simulink model "fullbridge1ph_igbt_model"  (R2026a)
settings: Solver=ode23t  StopTime=simStopTime
model workspace (MAT data in the model file):
  Cies_IGBT = 5.1e-09
  Cies_IGBT_nF = 5.1
  Cies_IGBT_pF = 5100
  Coes_IGBT = 1e-09
  Coes_IGBT_nF = 1
  Coes_IGBT_pF = 1000
  Cres_IGBT = 3e-10
  Cres_IGBT_nF = 0.3
  Cres_IGBT_pF = 300
  Eoff_sw = 0.0038
  Eon_sw = 0.009
  Eref_I_IGBT = 75
  Eref_T_IGBT = 125
  Eref_V_IGBT = 600
  Ic_VceSat = 75
  Ices = 0.005
  Tmeas_IGBT = 25
  VCE0_IGBT = 1.54
  VceSat = 3.85
  Vces_Ices = 1200
  VgeTh = 5.5
  Vge_VceSat = 15
  Vth = 5.5
  Vth_sw = 5.5
  rCE_IGBT = 0.0308
undefined symbols (not defined in the file): deadSamples, fout, fsw, ModIndex, Rload, Ts_ctrl, Vg
libraries: nesl_utility x28, fl_lib x27, ee_lib x15, simulink x1
(part 2 of 2)

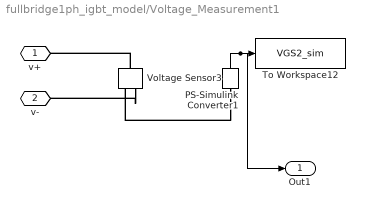
== system fullbridge1ph_igbt_model/Voltage_Measurement1 ==
  PS-Simulink Converter1 : nesl_utility/PS-Simulink Converter  PhysicalDomain=network_engine_domain  SubClassName=ps_output  LeftPortType=input  RightPortType=output  PseudoPeriodic=off  Frequencies=[]  VectorFormat=inherit  Unit=inherit  AffineConversion=off
  To Workspace12 : ToWorkspace  VariableName=VGS2_sim  SaveFormat=Timeseries  SampleTime=-1
  Voltage Sensor3 : fl_lib/Electrical/Electrical Sensors/Voltage Sensor
  v+ : PMIOPort  Side=Left
  v- : PMIOPort  Port=2  Side=Left
  Out1 : Outport
  wires:
  PS-Simulink Converter1/1 -> Out1/1, To Workspace12/1
  connections:
  Voltage Sensor3/RConn2 -- v-/RConn1
  PS-Simulink Converter1/LConn1 -- Voltage Sensor3/RConn1
  Voltage Sensor3/LConn1 -- v+/RConn1

== system fullbridge1ph_igbt_model/Voltage_Measurement2 ==
  PS-Simulink Converter1 : nesl_utility/PS-Simulink Converter  PhysicalDomain=network_engine_domain  SubClassName=ps_output  LeftPortType=input  RightPortType=output  PseudoPeriodic=off  Frequencies=[]  VectorFormat=inherit  Unit=inherit  AffineConversion=off
  To Workspace12 : ToWorkspace  VariableName=VGS1_sim  SaveFormat=Timeseries  SampleTime=-1
  Voltage Sensor3 : fl_lib/Electrical/Electrical Sensors/Voltage Sensor
  v+ : PMIOPort  Side=Left
  v- : PMIOPort  Port=2  Side=Left
  Out1 : Outport
  wires:
  PS-Simulink Converter1/1 -> Out1/1, To Workspace12/1
  connections:
  Voltage Sensor3/RConn2 -- v-/RConn1
  PS-Simulink Converter1/LConn1 -- Voltage Sensor3/RConn1
  Voltage Sensor3/LConn1 -- v+/RConn1

== system fullbridge1ph_igbt_model/Voltage_Measurement3 ==
  PS-Simulink Converter1 : nesl_utility/PS-Simulink Converter  PhysicalDomain=network_engine_domain  SubClassName=ps_output  LeftPortType=input  RightPortType=output  PseudoPeriodic=off  Frequencies=[]  VectorFormat=inherit  Unit=inherit  AffineConversion=off
  To Workspace12 : ToWorkspace  VariableName=VGS3_sim  SaveFormat=Timeseries  SampleTime=-1
  Voltage Sensor3 : fl_lib/Electrical/Electrical Sensors/Voltage Sensor
  v+ : PMIOPort  Side=Left
  v- : PMIOPort  Port=2  Side=Left
  wires:
  PS-Simulink Converter1/1 -> To Workspace12/1
  connections:
  Voltage Sensor3/RConn2 -- v-/RConn1
  PS-Simulink Converter1/LConn1 -- Voltage Sensor3/RConn1
  Voltage Sensor3/LConn1 -- v+/RConn1

== system fullbridge1ph_igbt_model/Voltage_Measurement4 ==
  PS-Simulink Converter1 : nesl_utility/PS-Simulink Converter  PhysicalDomain=network_engine_domain  SubClassName=ps_output  LeftPortType=input  RightPortType=output  PseudoPeriodic=off  Frequencies=[]  VectorFormat=inherit  Unit=inherit  AffineConversion=off
  To Workspace12 : ToWorkspace  VariableName=VGS4_sim  SaveFormat=Timeseries  SampleTime=-1
  Voltage Sensor3 : fl_lib/Electrical/Electrical Sensors/Voltage Sensor
  v+ : PMIOPort  Side=Left
  v- : PMIOPort  Port=2  Side=Left
  wires:
  PS-Simulink Converter1/1 -> To Workspace12/1
  connections:
  Voltage Sensor3/RConn2 -- v-/RConn1
  PS-Simulink Converter1/LConn1 -- Voltage Sensor3/RConn1
  Voltage Sensor3/LConn1 -- v+/RConn1

== system fullbridge1ph_igbt_model/Diode1_a/ID1_ToWorkspace ==
  PS-Simulink Converter1 : nesl_utility/PS-Simulink Converter  PhysicalDomain=network_engine_domain  SubClassName=ps_output  LeftPortType=input  RightPortType=output  PseudoPeriodic=off  Frequencies=[]  VectorFormat=inherit  Unit=inherit  AffineConversion=off
  To Workspace6 : ToWorkspace  VariableName=ID1_sim  SaveFormat=Timeseries  SampleTime=-1
  Conn1 : PMIOPort  Side=Right
  wires:
  PS-Simulink Converter1/1 -> To Workspace6/1
  connections:
  PS-Simulink Converter1/LConn1 -- Conn1/RConn1

== system fullbridge1ph_igbt_model/Diode1_a/Vd_ToWorkspace ==
  PS-Simulink Converter5 : nesl_utility/PS-Simulink Converter  PhysicalDomain=network_engine_domain  SubClassName=ps_output  LeftPortType=input  RightPortType=output  PseudoPeriodic=off  Frequencies=[]  VectorFormat=inherit  Unit=inherit  AffineConversion=off
  To Workspace12 : ToWorkspace  VariableName=VD1_sim  SaveFormat=Timeseries  SampleTime=-1
  y : PMIOPort  Side=Right
  wires:
  PS-Simulink Converter5/1 -> To Workspace12/1
  connections:
  y/RConn1 -- PS-Simulink Converter5/LConn1

== system fullbridge1ph_igbt_model/Diode1_b/ID1_ToWorkspace ==
  PS-Simulink Converter1 : nesl_utility/PS-Simulink Converter  PhysicalDomain=network_engine_domain  SubClassName=ps_output  LeftPortType=input  RightPortType=output  PseudoPeriodic=off  Frequencies=[]  VectorFormat=inherit  Unit=inherit  AffineConversion=off
  To Workspace6 : ToWorkspace  VariableName=ID3_sim  SaveFormat=Timeseries  SampleTime=-1
  Conn1 : PMIOPort  Side=Right
  wires:
  PS-Simulink Converter1/1 -> To Workspace6/1
  connections:
  PS-Simulink Converter1/LConn1 -- Conn1/RConn1

== system fullbridge1ph_igbt_model/Diode1_b/Vd_ToWorkspace ==
  PS-Simulink Converter5 : nesl_utility/PS-Simulink Converter  PhysicalDomain=network_engine_domain  SubClassName=ps_output  LeftPortType=input  RightPortType=output  PseudoPeriodic=off  Frequencies=[]  VectorFormat=inherit  Unit=inherit  AffineConversion=off
  To Workspace12 : ToWorkspace  VariableName=VD3_sim  SaveFormat=Timeseries  SampleTime=-1
  y : PMIOPort  Side=Right
  wires:
  PS-Simulink Converter5/1 -> To Workspace12/1
  connections:
  y/RConn1 -- PS-Simulink Converter5/LConn1

== system fullbridge1ph_igbt_model/Diode2_a/ID_ToWorkspace ==
  PS-Simulink Converter8 : nesl_utility/PS-Simulink Converter  PhysicalDomain=network_engine_domain  SubClassName=ps_output  LeftPortType=input  RightPortType=output  PseudoPeriodic=off  Frequencies=[]  VectorFormat=inherit  Unit=inherit  AffineConversion=off
  To Workspace6 : ToWorkspace  VariableName=ID2_sim  SaveFormat=Timeseries  SampleTime=-1
  y : PMIOPort  Side=Left
  wires:
  PS-Simulink Converter8/1 -> To Workspace6/1
  connections:
  y/RConn1 -- PS-Simulink Converter8/LConn1

== system fullbridge1ph_igbt_model/Diode2_a/Vd2_ToWorkspace ==
  PS-Simulink Converter7 : nesl_utility/PS-Simulink Converter  PhysicalDomain=network_engine_domain  SubClassName=ps_output  LeftPortType=input  RightPortType=output  PseudoPeriodic=off  Frequencies=[]  VectorFormat=inherit  Unit=inherit  AffineConversion=off
  To Workspace12 : ToWorkspace  VariableName=VD2_sim  SaveFormat=Timeseries  SampleTime=-1
  u : PMIOPort  Side=Left
  wires:
  PS-Simulink Converter7/1 -> To Workspace12/1
  connections:
  u/RConn1 -- PS-Simulink Converter7/LConn1

== system fullbridge1ph_igbt_model/Diode2_b/ID_ToWorkspace ==
  PS-Simulink Converter8 : nesl_utility/PS-Simulink Converter  PhysicalDomain=network_engine_domain  SubClassName=ps_output  LeftPortType=input  RightPortType=output  PseudoPeriodic=off  Frequencies=[]  VectorFormat=inherit  Unit=inherit  AffineConversion=off
  To Workspace6 : ToWorkspace  VariableName=ID4_sim  SaveFormat=Timeseries  SampleTime=-1
  y : PMIOPort  Side=Left
  wires:
  PS-Simulink Converter8/1 -> To Workspace6/1
  connections:
  y/RConn1 -- PS-Simulink Converter8/LConn1

== system fullbridge1ph_igbt_model/Diode2_b/Vd2_ToWorkspace ==
  PS-Simulink Converter7 : nesl_utility/PS-Simulink Converter  PhysicalDomain=network_engine_domain  SubClassName=ps_output  LeftPortType=input  RightPortType=output  PseudoPeriodic=off  Frequencies=[]  VectorFormat=inherit  Unit=inherit  AffineConversion=off
  To Workspace12 : ToWorkspace  VariableName=VD4_sim  SaveFormat=Timeseries  SampleTime=-1
  u : PMIOPort  Side=Left
  wires:
  PS-Simulink Converter7/1 -> To Workspace12/1
  connections:
  u/RConn1 -- PS-Simulink Converter7/LConn1

== matlab function fullbridge1ph_igbt_model/MATLAB Function1 ==
  data: G3raw input; G3 output; G4raw input; Ndead input; G4 output
function [G3, G4] = deadtime_G3G4(G3raw, G4raw, Ndead)

persistent G3_state G4_state cnt3 cnt4

if isempty(G3_state)
    G3_state = false;
    G4_state = false;
    cnt3 = 0;
    cnt4 = 0;
end

G3raw = logical(G3raw);
G4raw = logical(G4raw);
Ndead = max(0, round(Ndead));

if G3raw && G4raw
    G3_state = false;
    G4_state = false;
    cnt3 = 0;
    cnt4 = 0;

elseif G3raw
    G4_state = false;
    cnt4 = 0;

    if cnt3 >= Ndead
        G3_state = true;
    else
        G3_state = false;
        cnt3 = cnt3 + 1;
    end

elseif G4raw
    G3_state = false;
    cnt3 = 0;

    if cnt4 >= Ndead
        G4_state = true;
    else
        G4_state = false;
        cnt4 = cnt4 + 1;
    end

else
    G3_state = false;
    G4_state = false;
    cnt3 = 0;
    cnt4 = 0;
end

G3 = G3_state;
G4 = G4_state;

end

== matlab function fullbridge1ph_igbt_model/MATLAB Function ==
  data: G1raw input; G1 output; G2raw input; Ndead input; G2 output
function [G1, G2] = deadtime_G1G2(G1raw, G2raw, Ndead)

persistent G1_state G2_state cnt1 cnt2

if isempty(G1_state)
    G1_state = false;
    G2_state = false;
    cnt1 = 0;
    cnt2 = 0;
end

G1raw = logical(G1raw);
G2raw = logical(G2raw);
Ndead = max(0, round(Ndead));

if G1raw && G2raw
    G1_state = false;
    G2_state = false;
    cnt1 = 0;
    cnt2 = 0;

elseif G1raw
    G2_state = false;
    cnt2 = 0;

    if cnt1 >= Ndead
        G1_state = true;
    else
        G1_state = false;
        cnt1 = cnt1 + 1;
    end

elseif G2raw
    G1_state = false;
    cnt1 = 0;

    if cnt2 >= Ndead
        G2_state = true;
    else
        G2_state = false;
        cnt2 = cnt2 + 1;
    end

else
    G1_state = false;
    G2_state = false;
    cnt1 = 0;
    cnt2 = 0;
end

G1 = G1_state;
G2 = G2_state;

end
